simulink model "H175_PANKL_V1a_controlled_R2022b"  (R2022b)
settings: Solver=ode15s  StartTime=0.0  StopTime=22136  RelTol=1e-3  AbsTol=1e-3
PreLoadFcn:
  | omega_TLU = [1000, 1500, 2000, 2500, 3000, 3500];
  | beta_TLU = linspace(0,1,7);
  | 
  | mdot_TLU = [0.1377    0.1304    0.1187    0.1029    0.0854    0.0658    0.0437
  |     0.2310    0.2183    0.1978    0.1688    0.1400    0.1118    0.0750
  |     0.3298    0.3208    0.2987    0.2677    0.2256    0.1774    0.1194
  |     0.4520    0.4260    0.3825    0.3308    0.2745    0.2227    0.1655
  |     0.5542    0.5353    0.4781    0.4230    0.3477    0.2897    0.2211
  |     0.6197    0.5805    0.5198    0.4516    0.3971    0.3555    0.2825];
  | 
  | eta_TLU = [0.7905    0.8025    0.7998    0.7972    0.7932    0.7882    0.7827
  |     0.7993    0.8239    0.8350    0.8379    0.8197    0.8000    0.7809
  |     0.8011    0.8374    0.8632    0.8827    0.8749    0.8394    0.7948
  |     0.8072    0.8520    0.8814    0.9000    0.8676    0.8356    0.7971
  |     0.8076    0.8271    0.8608    0.8766    0.8529    0.8329    0.7992
  |     0.7949    0.8131    0.8296    0.8243    0.8170    0.8085    0.7972];
  | 
  | pr_TLU = [1.0912    1.1795    1.2293    1.2662    1.2928    1.3108    1.3151
  |     1.1484    1.3081    1.3958    1.4707    1.5136    1.5380    1.5456
  |     1.2830    1.4539    1.5943    1.7042    1.7973    1.8582    1.8799
  |     1.5180    1.8034    1.9693    2.0899    2.1662    2.2027    2.2182
  |     1.8359    2.0956    2.3359    2.4668    2.5687    2.6106    2.6224
  |     2.3061    2.6623    2.8585    2.9837    3.0443    3.0714    3.0869];
values from neighbouring files (symbols this model uses):
  P64_omega_TLU = [44762 68636 92509 110414 125335 137271 146224]    [All_Properties.mat]    (also in PANKL_CMP.mat = [44762 68636 92509 110414 125335 137271 146224 155176.0695 1)
libraries: fl_lib x101, nesl_utility x76, SimscapeFluids_lib x5, slpidlib x3
(part 2 of 4)

== system H175_PANKL_V1a_controlled_R2022b/Coolant Tank2 ==
  Coolant Volume : fl_lib/Thermal Liquid/Elements/Translational Mechanical Converter (TL)  mech_orientation=foundation.enum.MechOrientationTranslational.Positive  displacement_spec=foundation.enum.DisplacementSpec.Calculate  x0=x_init m  interface_area=A m^2  dead_volume=A * 0.001 m^3  environment_spec=foundation.enum.pressure_spec.atmospheric  environment_pressure=0.101325 MPa  dynamic_compressibility=simscape.enum.onoff.off  p0=env_p MPa  T0=20 degC
      settings: InternalSimscapePortConfiguration="{\"Bottom\":[],\"Left\":[{\"id\":\"A\",\"label\":\"A\",\"type\":\"foundation.thermal_liquid.thermal_liquid\"},{\"id\":\"C\",\"label\":\"C\",\"type\":\"foundation.mechanical.translational.translational\"},{\"id\":\"H\",\"label\":\"H\",\"type\":\"foundation.thermal.thermal\"}],\"Right\":[{\"id\":\"R\",\"label\":\"R\",\"type\":\"foundation.mechanical.translational.translational\"}],\"Top\":[]}"
  Mechanical Translational Reference : fl_lib/Mechanical/Translational Elements/Mechanical Translational Reference
  Perfect Insulator : fl_lib/Thermal/Thermal Elements/Perfect Insulator  T_specify=off  T_priority=None  T=0 K  T_nominal_specify=off  T_nominal_unit=K  T_nominal_value=1
  Translational Free End : fl_lib/Mechanical/Translational Elements/Translational Free End  v_specify=off  v_priority=None  v=0 m/s  v_nominal_specify=off  v_nominal_unit=m/s  v_nominal_value=1
      settings: InternalSimscapePortConfiguration="{\"Bottom\":[],\"Left\":[{\"id\":\"V\",\"label\":\"\",\"type\":\"foundation.mechanical.translational.translational\"}],\"Right\":[],\"Top\":[]}"
  T : PMIOPort  Side=Right
  connections:
  Coolant Volume/LConn1 -- T/RConn1
  Mechanical Translational Reference/LConn1 -- Coolant Volume/LConn2
  Translational Free End/LConn1 -- Coolant Volume/RConn1
  Perfect Insulator/LConn1 -- Coolant Volume/LConn3
